simulink model "Book6142"  (R2019b)
settings: Solver=ode4  StartTime=0  StopTime=20  FixedStep=0.001  RelTol=1e-3
settings Model: Creator=user  LastModifiedBy=xyh

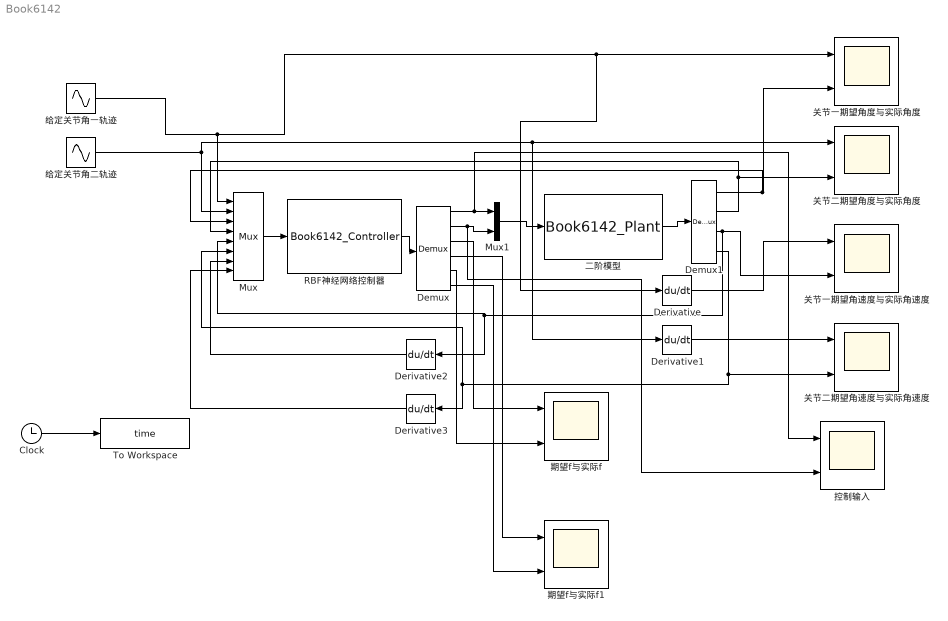
== system Book6142 ==
  Clock : Clock
  Demux : Demux  Outputs=6
  Demux1 : Demux
  Derivative{,1..3} (4 alike) : Derivative
  Mux : Mux  Inputs=8
  Mux1 : Mux  Inputs=2
  RBF神经网络控制器 : S-Function  FunctionName=Book6142_Controller  SFunctionDeploymentMode=off  EnableBusSupport=off
  To Workspace : ToWorkspace  VariableName=time  SaveFormat=Timeseries  SampleTime=-1
  二阶模型 : S-Function  FunctionName=Book6142_Plant  SFunctionDeploymentMode=off  EnableBusSupport=off
  关节一期望角度与实际角度 : Scope  NumInputPorts=2
  关节一期望角速度与实际角速度 : Scope  NumInputPorts=2
  关节二期望角度与实际角度 : Scope  NumInputPorts=2
  关节二期望角速度与实际角速度 : Scope  NumInputPorts=2
  控制输入 : Scope  NumInputPorts=2
  期望f与实际f : Scope  NumInputPorts=2
  期望f与实际f1 : Scope  NumInputPorts=2
  给定关节角一轨迹 : Sin  Amplitude=0.2  Bias=1  Frequency=0.5*pi  SampleTime=0
  给定关节角二轨迹 : Sin  Amplitude=-0.2  Bias=1  Frequency=0.5*pi  Phase=pi/2  SampleTime=0
  wires:
  二阶模型/1 -> Demux1/1
  给定关节角一轨迹/1 -> Derivative/1, 关节一期望角度与实际角度/1, Mux/1
  Mux/1 -> RBF神经网络控制器/1
  Clock/1 -> To Workspace/1
  给定关节角二轨迹/1 -> Mux/2, 关节二期望角度与实际角度/1, Derivative1/1
  Derivative/1 -> 关节一期望角速度与实际角速度/1
  Derivative1/1 -> 关节二期望角速度与实际角速度/1
  Demux1/1 -> Mux/3, 关节一期望角度与实际角度/2
  Demux1/2 -> Mux/4, 关节二期望角度与实际角度/2
  Demux1/3 -> Derivative2/1, Mux/5, 关节一期望角速度与实际角速度/2
  Demux1/4 -> 关节二期望角速度与实际角速度/2, Derivative3/1, Mux/6
  RBF神经网络控制器/1 -> Demux/1
  Derivative2/1 -> Mux/7
  Derivative3/1 -> Mux/8
  Demux/1 -> 控制输入/1, Mux1/1
  Demux/2 -> 控制输入/2, Mux1/2
  Mux1/1 -> 二阶模型/1
  Demux/3 -> 期望f与实际f/1
  Demux/5 -> 期望f与实际f/2
  Demux/4 -> 期望f与实际f1/1
  Demux/6 -> 期望f与实际f1/2
